simulink model "Halfadder_Model"  (R2024b)
settings: Solver=VariableStepAuto  StartTime=0.0  StopTime=10.0  RelTol=1e-3
libraries: NSA_DEVS_SINKS x4, NSA_DEVS_LOGISTICS x2, NSA_DEVS_SOURCES x2, NSA_DEVS_DIGITAL_LOGIC x1
settings Model: Creator=david  LastModifiedBy=peter
settings RTWCC: GPUComputeCapability=3.5

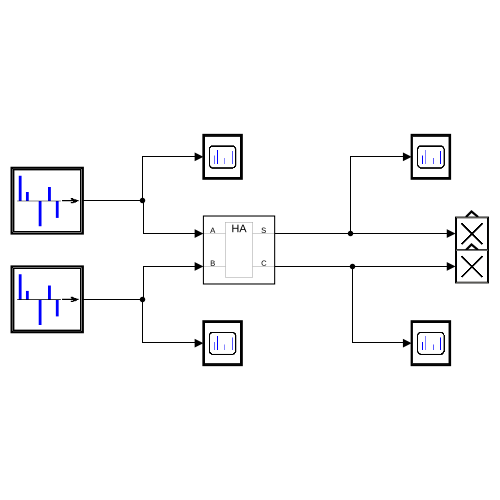
[thumbnail: Simulink's stored preview of the top-level diagram]
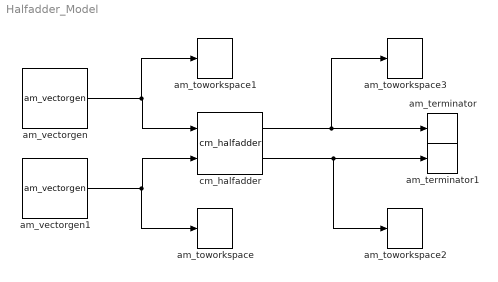
== system Halfadder_Model ==
  am_terminator : NSA_DEVS_LOGISTICS/am_terminator  tau=[0,1]  debug=0
      settings: SourceProductName=Logistics
  am_terminator1 : NSA_DEVS_LOGISTICS/am_terminator  tau=[0,1]  debug=0
      settings: SourceProductName=Logistics
  am_toworkspace : NSA_DEVS_SINKS/am_toworkspace  varname="\"gen2Out\""  t0=0  format="\"vector\""  tau=[0,5]  debug=0
      settings: SourceProductName=Sinks
  am_toworkspace1 : NSA_DEVS_SINKS/am_toworkspace  varname="\"gen1Out\""  t0=0  format="\"vector\""  tau=[0,5]  debug=0
      settings: SourceProductName=Sinks
  am_toworkspace2 : NSA_DEVS_SINKS/am_toworkspace  varname="\"hacOut\""  t0=0  format="\"vector\""  tau=[0,5]  debug=0
      settings: SourceProductName=Sinks
  am_toworkspace3 : NSA_DEVS_SINKS/am_toworkspace  varname="\"hasOut\""  t0=0  format="\"vector\""  tau=[0,5]  debug=0
      settings: SourceProductName=Sinks
  am_vectorgen : NSA_DEVS_SOURCES/am_vectorgen  tvec="[1,    2,   3,   6,   7,   8,  10]"  yvec="[\"0\", \"1\", \"0\", \"1\", \"0\", \"1\", \"0\"]"  tau=[0,1]  debug=0
      settings: SourceProductName=Sources
  am_vectorgen1 : NSA_DEVS_SOURCES/am_vectorgen  tvec="[1,    4,   5,   6,   7,   9,  10]"  yvec="[\"0\", \"1\", \"0\", \"1\", \"0\", \"1\", \"0\"]"  tau=[0,1]  debug=0
      settings: SourceProductName=Sources
  cm_halfadder : NSA_DEVS_DIGITAL_LOGIC/cm_halfadder  tau=[0,1]  debug=0
      settings: SourceProductName=Logic
  wires:
  am_vectorgen/1 -> am_toworkspace1/1, cm_halfadder/1
  cm_halfadder/2 -> am_toworkspace2/1, am_terminator1/1
  cm_halfadder/1 -> am_toworkspace3/1, am_terminator/1
  am_vectorgen1/1 -> am_toworkspace/1, cm_halfadder/2
